simulink model "req19B"  (R2019a)
settings: Solver=FixedStepAuto  StartTime=0.0  StopTime=100  RelTol=1e-3
settings Model: Creator=e40014285  LastModifiedBy=e40014285
settings ConfigComp: CovScope=ReferencedModels  CovIncludeTopModel=off  CovHTMLOptions=-sRT=1 -sVT=0 -aTS=1 -bRG=1 -bTC=1 -hTR=0 -nFC=0 -nFD=1 -scm=1 -bcm=1 -xEv=0 -xEM=0  CovHtmlReporting=on  CovCumulativeReport=on  DVMaxProcessTime=6000  DVModelCoverageObjectives=EnhancedMCDC  DVTestSuiteOptimization=Auto  DVDetectOutOfBounds=on  DVReportPDFFormat=on  DVRebuildModelRepresentation=Always

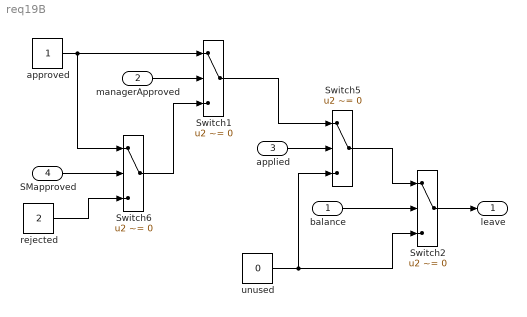
== system req19B ==
  balance : Inport
  managerApproved : Inport  Port=2
  applied : Inport  Port=3
  SMapproved : Inport  Port=4
  Switch{1..2,5..6} (4 alike) : Switch  Criteria=u2 ~= 0
  approved : Constant
  rejected : Constant  Value=2
  unused : Constant  Value=0
  leave : Outport
  wires:
  balance/1 -> Switch2/2
  Switch2/1 -> leave/1
  Switch5/1 -> Switch2/1
  unused/1 -> Switch5/3, Switch2/3
  applied/1 -> Switch5/2
  SMapproved/1 -> Switch6/2
  approved/1 -> Switch6/1, Switch1/1
  managerApproved/1 -> Switch1/2
  Switch1/1 -> Switch5/1
  Switch6/1 -> Switch1/3
  rejected/1 -> Switch6/3
